simulink library "Susp_AxleTA4Watts"  (R2025b)
settings: Solver=VariableStepAuto  StartTime=0.0  StopTime=10.0  RelTol=1e-3
undefined symbols (not defined in the file): Axle1D, AxleIn, Init, RaceFix, RaceSpin, Susp, Visual, X, Y, Z
libraries: sm_lib x57, Susp_Components x7, Suspension_Utilities x4, Linkage_Shock x2, fl_lib x2, nesl_utility x2, Linkage_Spring x2, Linkage_Bumpstop x1
(part 1 of 3)
Description:
  | Component of Simscape Vehicle Templates Library
  | 
  | Copyright 2018-2025 The MathWorks, Inc.
settings Model: Creator=mwalker  LastModifiedBy=smiller
settings SolverCC: AlgebraicLoopSolver=TrustRegion
settings DataIOCC: ReturnWorkspaceOutputs=off
settings DebuggingCC: UnconnectedInputMsg=warning  UnconnectedOutputMsg=warning  UnconnectedLineMsg=warning  ArithmeticOperatorsInVariantConditions=warning
settings ModelReferenceCC: EnableRefExpFcnMdlSchedulingChecks=on
settings SFSimCC: CustomCodeUndefinedFunction=UseInterfaceOnly
settings RTWCC: GPUComputeCapability=3.5

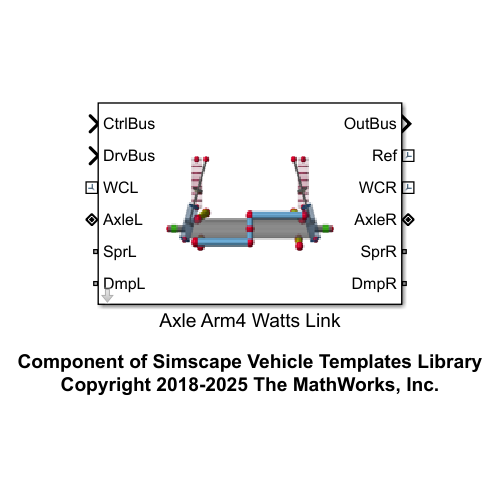
[thumbnail: Simulink's stored preview of the top-level diagram]
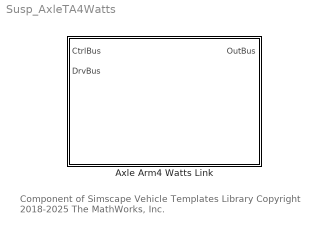
== system Susp_AxleTA4Watts ==
  note: Component of Simscape Vehicle Templates Library
      | Copyright 2018-2025 The MathWorks, Inc.
  Axle Arm4 Watts Link : Subsystem  VariantControl=LiveAxle  mask(Rigid Axle 4 Trailing Arm Watts Link Suspension){Init=Init.Axle2, hp_damper_top=Susp.AxleTA4Watts.Damper.sTop.Value, hp_damper_bot=Susp.AxleTA4Watts.Damper.sBottom.Value, hp_spring_top=Susp.AxleTA4Watts.Spring.sTop.Value, hp_spring_bot=Susp.AxleTA4Watts.Spring.sBottom.Value, hp_ua_body=Susp.AxleTA4Watts.TrailingArmUpper.sBody.Value, hp_ua_axle=Susp.AxleTA4Watts.TrailingArmUpper.sAxle.Value, hp_la_body=Susp.AxleTA4Watts.TrailingArmLower.sBody.Value, hp_la_axle=Susp.AxleTA4Watts.TrailingArmLower.sAxle.Value, hp_wattsu_body=Susp.AxleTA4Watts.WattsLinkUpper.sBody.Value, hp_wattsu_pivot=Susp.AxleTA4Watts.WattsLinkUpper.sPivot.Value, hp_wattsl_body=Susp.AxleTA4Watts.WattsLinkLower.sBody.Value, hp_wattsl_pivot=Susp.AxleTA4Watts.WattsLinkLower.sPivot.Value, hp_wattsp_axle=Susp.AxleTA4Watts.WattsLinkPivot.sAxle.Value, hp_axle_cg=Susp.AxleTA4Watts.Axle.sCG.Value, hp_whl_ctr=Susp.AxleTA4Watts.Axle.sWheelCentre.Value, hp_chassis_bumpstop=Susp.AxleTA4Watts.Bumpstop.sChassis.Value, hp_axle_bumpstop=Susp.AxleTA4Watts.Bumpstop.sAxle.Value, axle_mass=Susp.AxleTA4Watts.Axle.m.Value, stub_axle_len=Susp.AxleTA4Watts.StubAxle.xAxle.Value, stub_axle_mass=Susp.AxleTA4Watts.StubAxle.m.Value, axle_whlc_to_bearing=Susp.AxleTA4Watts.Axle.xWCtoBearing.Value, ua_mass=Susp.AxleTA4Watts.TrailingArmUpper.m.Value, la_mass=Susp.AxleTA4Watts.TrailingArmLower.m.Value, wattsu_mass=Susp.AxleTA4Watts.WattsLinkUpper.m.Value, wattsl_mass=Susp.AxleTA4Watts.WattsLinkLower.m.Value, wattsp_mass=Susp.AxleTA4Watts.WattsLinkLower.m.Value, clr_conn_rod=Visual.hp.clr, opc_conn_rod=Visual.hp.opc, size_conn_rod=Visual.hp.rad, clr_rod=Visual.UpperArm.clr, opc_rod=Visual.part.opc, radius_rod=Visual.UpperArm.rad, clr_link=Visual.Pushrod.clr, opc_link=Visual.part.opc, radius_link=Visual.Pushrod.rad, axle_clr=[0.5 0.5 0.5], axle_opc=Visual.part.opc, clr_stub_axle=Visual.Axle.clr, opc_stub_axle=Visual.part.opc, rad_stub_axle=Visual.Axle.rad, shock_pist_mass=Susp.AxleTA4Watts.Damper.mPiston.Value, shock_cyl_mass=Susp.AxleTA4Watts.Damper.mCylinder.Value, shock_xmax=Susp.AxleTA4Watts.Endstop.xMax.Value, shock_xmin=Susp.AxleTA4Watts.Endstop.xMin.Value, spring_mass=Susp.AxleTA4Watts.Spring.m.Value, Bumpstop_Type=Susp.AxleTA4Watts.Bumpstop.class.Value, bumpstop_height=Susp.AxleTA4Watts.Bumpstop.xHeight.Value, bumpstop_k=Susp.AxleTA4Watts.Bumpstop.K.Value, bumpstop_d=Susp.AxleTA4Watts.Bumpstop.d.Value, bumpstop_xTrans=Susp.AxleTA4Watts.Bumpstop.xTransition.Value, bumpstop_ptcld=Susp.AxleTA4Watts.Bumpstop.sPointCloud.Value}
      mask prompts: Init "Initial Wheel Speed (rad/s)"; hp_damper_top "HP Damper Top [xyz] (m)"; hp_damper_bot "Damper Bottom [xyz] (m)"; hp_spring_top "HP Spring Top [xyz] (m)"; hp_spring_bot "HP Spring Bottom [xyz] (m)"; hp_ua_body "HP Trailing Arm Upper to Body [xyz] (m)"; hp_ua_axle "HP Trailing Arm Upper to Axle [xyz] (m)"; hp_la_body "HP Trailing Arm Lower to Body [xyz] (m)"; hp_la_axle "HP Trailing Arm Lower to Axle [xyz] (m)"; hp_wattsu_body "HP Watts Link Upper to Body [xyz] (m)"; hp_wattsu_pivot "HP Watts Link Upper to Pivot [xyz] (m)"; hp_wattsl_body "HP Watts Link Lower to Body [xyz] (m)"; hp_wattsl_pivot "HP Watts Link Lower to Pivot [xyz] (m)"; hp_wattsp_axle "HP Watts Link Pivot to Axle [xyz] (m)"; hp_axle_cg "HP Axle CG [xyz] (m)"; hp_whl_ctr "HP Wheel Center [xyz] (m)"; hp_chassis_bumpstop "HP Bumpstop Chassis [xyz] (m)"; hp_axle_bumpstop "HP Bumpstop Axle [xyz] (m)"; axle_mass "Axle Mass (kg)"; stub_axle_len "Stub Axle Length (m)"; stub_axle_mass "Stub Axle Mass (kg)"; axle_whlc_to_bearing "Distance Wheel Ctr to Bearing (m)"; ua_mass "Trailing Arm Upper Mass (kg)"; la_mass "Trailing Arm Lower Mass (kg)"; wattsu_mass "Watts Link Upper Mass (kg)"; wattsl_mass "Watts Link Lower Mass (kg)"; wattsp_mass "Watts Link Pivot Mass (kg)"; shock_pist_mass "Piston Mass (kg)"; shock_cyl_mass "Cylinder Mass (kg)"; shock_xmax "Upper Limit Bumpstop (m)"; shock_xmin "Lower Limit Bumpstop (m)"; spring_mass "Spring Mass (kg)"; Bumpstop_Type "Type"; bumpstop_height "Height (m)"; bumpstop_k "Stiffness (N/m)"; bumpstop_d "Damping (N/(m/s))"; bumpstop_xTrans "Transition Depth (m)"; bumpstop_ptcld "Point Cloud [xyz] (m)"
      mask help: Models a rigid axle connected to the chassis by four trailing arms and a Watts linkage.The displacement of the springs and dampers are modeled here and the forces are modeled in a separate subsystem.
      mask TypeOptions hp_damper_top: DamperL/hp_spr_top | DamperR/hp_spr_top | Hardpoints/hp_damper_top
      mask TypeOptions hp_damper_bot: Axle/hp_damper_bot | DamperL/hp_spr_bot | DamperR/hp_spr_bot
      mask TypeOptions hp_spring_top: Hardpoints/hp_spring_top | SpringL/hp_spr_top | SpringR/hp_spr_top
      mask TypeOptions hp_spring_bot: Axle/hp_spring_bot | SpringL/hp_spr_bot | SpringR/hp_spr_bot
      mask TypeOptions hp_ua_body:
      | Hardpoints/hp_ua_body | Trailing
      | UpperL/hp_in | Trailing
      | UpperR/hp_in
      mask TypeOptions hp_ua_axle:
      | Axle/hp_ua_axle | Trailing
      | UpperL/hp_out | Trailing
      | UpperR/hp_out
      mask TypeOptions hp_la_body:
      | Hardpoints/hp_la_body | Trailing
      | LowerL/hp_in | Trailing
      | LowerR/hp_in
      mask TypeOptions hp_la_axle:
      | Axle/hp_la_axle | Trailing
      | LowerL/hp_out | Trailing
      | LowerR/hp_out
      mask TypeOptions hp_wattsu_body: Hardpoints/hp_wattsu_body | Watts/hp_wattsu_body
      mask TypeOptions hp_wattsu_pivot: Watts/hp_wattsu_pivot
      mask TypeOptions hp_wattsl_body: Hardpoints/hp_wattsl_body | Watts/hp_wattsl_body
      mask TypeOptions hp_wattsl_pivot: Watts/hp_wattsl_pivot
      mask TypeOptions hp_wattsp_axle: Axle/hp_wattsp_axle | Watts/hp_wattsp_axle
      mask TypeOptions hp_axle_cg: Axle/hp_axle_cg
      mask TypeOptions hp_whl_ctr: Axle/hp_whl_ctr
      mask TypeOptions hp_chassis_bumpstop: Hardpoints/hp_chassis_bumpstop
      mask TypeOptions hp_axle_bumpstop: Axle/hp_axle_bumpstop
      mask TypeOptions axle_mass: Axle/axle_mass
      mask TypeOptions stub_axle_len: Stub Axle L/stub_axle_len | Stub Axle R/stub_axle_len
      mask TypeOptions stub_axle_mass: Stub Axle L/stub_axle_mass | Stub Axle R/stub_axle_mass
      mask TypeOptions axle_whlc_to_bearing: Axle/axle_whlc_to_bearing
      mask TypeOptions ua_mass:
      | Trailing
      | UpperL/rod_mass | Trailing
      | UpperR/rod_mass
      mask TypeOptions la_mass:
      | Trailing
      | LowerL/rod_mass | Trailing
      | LowerR/rod_mass
      mask TypeOptions wattsu_mass: Watts/wattsu_mass
      mask TypeOptions wattsl_mass: Watts/wattsl_mass
      mask TypeOptions wattsp_mass: Watts/wattsp_mass
      mask TypeOptions clr_conn_rod:
      | Trailing
      | LowerL/clr_conn_rod | Trailing
      | LowerR/clr_conn_rod | Trailing
      | UpperL/clr_conn_rod | Trailing
      | UpperR/clr_conn_rod | Watts/clr_conn_rod
      mask TypeOptions opc_conn_rod:
      | Trailing
      | LowerL/opc_conn_rod | Trailing
      | LowerR/opc_conn_rod | Trailing
      | UpperL/opc_conn_rod | Trailing
      | UpperR/opc_conn_rod | Watts/opc_conn_rod
      mask TypeOptions size_conn_rod:
      | Trailing
      | LowerL/size_conn_rod | Trailing
      | LowerR/size_conn_rod | Trailing
      | UpperL/size_conn_rod | Trailing
      | UpperR/size_conn_rod | Watts/size_conn_rod
      mask TypeOptions clr_rod:
      | Trailing
      | LowerL/clr_rod | Trailing
      | LowerR/clr_rod | Trailing
      | UpperL/clr_rod | Trailing
      | UpperR/clr_rod
      mask TypeOptions opc_rod:
      | Trailing
      | LowerL/opc_rod | Trailing
      | LowerR/opc_rod | Trailing
      | UpperL/opc_rod | Trailing
      | UpperR/opc_rod
      mask TypeOptions radius_rod:
      | Trailing
      | LowerL/radius_rod | Trailing
      | LowerR/radius_rod | Trailing
      | UpperL/radius_rod | Trailing
      | UpperR/radius_rod
      mask TypeOptions clr_link: Watts/clr_link
      mask TypeOptions opc_link: Watts/opc_link
      mask TypeOptions radius_link: Watts/radius_link
      mask TypeOptions axle_clr: Axle/axle_clr
      mask TypeOptions axle_opc: Axle/axle_opc
      mask TypeOptions clr_stub_axle: Stub Axle L/clr_stub_axle | Stub Axle R/clr_stub_axle
      mask TypeOptions opc_stub_axle: Stub Axle L/opc_stub_axle | Stub Axle R/opc_stub_axle
      mask TypeOptions rad_stub_axle: Stub Axle L/rad_stub_axle | Stub Axle R/rad_stub_axle
      mask TypeOptions shock_pist_mass: DamperL/shock_pist_mass | DamperR/shock_pist_mass
      mask TypeOptions shock_cyl_mass: DamperL/shock_cyl_mass | DamperR/shock_cyl_mass
      mask TypeOptions shock_xmax: DamperL/up_lim_bumpstop | DamperR/up_lim_bumpstop
      mask TypeOptions shock_xmin: DamperL/low_lim_bumpstop | DamperR/low_lim_bumpstop
      mask TypeOptions spring_mass: SpringL/spring_mass | SpringR/spring_mass
      mask DialogControl cont_hp Prompt: Hardpoints, Axes
      mask DialogControl cont_parts Prompt: Parts
      mask DialogControl Container7 Prompt: Visualization
      mask DialogControl text_clr Prompt: Color [RGB]
      mask DialogControl text_opc Prompt: Opac. (0-1)
      mask DialogControl text_size Prompt: Size (m)
      mask DialogControl text_conn Prompt: Connections
      mask DialogControl text_arms Prompt: Arms
      mask DialogControl text_links Prompt: Links
      mask DialogControl text_axle Prompt: Axle
      mask DialogControl text_axle_size Prompt: <derived>
      mask DialogControl text_Stub_Axle Prompt: Stub Axle
      mask DialogControl cont_shock Prompt: Shock
      mask DialogControl cont_bumpstop Prompt: Bumpstop
      mask Display: image('sm_car_vehicle_susp_axleta4watts_IMAGE.png');
